simulink model "prob7_large_model"  (R2013a)
settings: Solver=ode45  StartTime=0.0  StopTime=0.5  RelTol=1e-3
libraries: fl_lib x10, nesl_utility x4
settings Model: Creator=Suddenlink  LastModifiedBy=Suddenlink

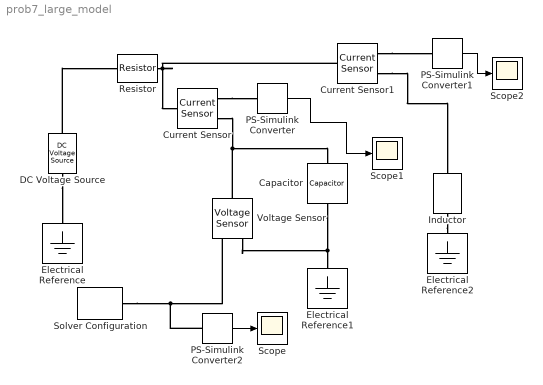
== system prob7_large_model ==
  Capacitor : fl_lib/Electrical/Electrical Elements/Capacitor  c=1e-6 F  v0=0 V  r=1e-6 Ohm  g=0 1/Ohm  i_Log=off  v_Log=off  vc_Log=off  LocalVarNames=|i|v|vc  LocalVarDescs=|i|v|Internal variable for voltage across capacitor term  LocalVarLogging=[0 0 0]
  Current Sensor : fl_lib/Electrical/Electrical Sensors/Current Sensor  i1_Log=off  v1_Log=off  LocalVarNames=|i1|v1  LocalVarDescs=|i1|v1  LocalVarLogging=[0 0]
  Current Sensor1 : fl_lib/Electrical/Electrical Sensors/Current Sensor  i1_Log=off  v1_Log=off  LocalVarNames=|i1|v1  LocalVarDescs=|i1|v1  LocalVarLogging=[0 0]
  DC Voltage Source : fl_lib/Electrical/Electrical Sources/DC Voltage Source  v0=1 V  i_Log=off  v_Log=off  LocalVarNames=|i|v  LocalVarDescs=|i|v  LocalVarLogging=[0 0]
  Electrical Reference : fl_lib/Electrical/Electrical Elements/Electrical Reference  i_Log=off  LocalVarNames=|i  LocalVarDescs=|i  LocalVarLogging=0
  Electrical Reference1 : fl_lib/Electrical/Electrical Elements/Electrical Reference  i_Log=off  LocalVarNames=|i  LocalVarDescs=|i  LocalVarLogging=0
  Electrical Reference2 : fl_lib/Electrical/Electrical Elements/Electrical Reference  i_Log=off  LocalVarNames=|i  LocalVarDescs=|i  LocalVarLogging=0
  Inductor : fl_lib/Electrical/Electrical Elements/Inductor  l=1e-6 H  i0=0 A  r=0 Ohm  g=1e-9 1/Ohm  i_Log=off  v_Log=off  i_L_Log=off  LocalVarNames=|i|v|i_L  LocalVarDescs=|i|v|Internal variable for current through inductor term  LocalVarLogging=[0 0 0]
  PS-Simulink Converter : nesl_utility/PS-Simulink Converter  PhysicalDomain=network_engine_domain  SubClassName=ps_output  LeftPortType=input  RightPortType=output  PseudoPeriodic=off  Frequencies=[]  Unit=1  AffineConversion=off
  PS-Simulink Converter1 : nesl_utility/PS-Simulink Converter  PhysicalDomain=network_engine_domain  SubClassName=ps_output  LeftPortType=input  RightPortType=output  PseudoPeriodic=off  Frequencies=[]  Unit=1  AffineConversion=off
  PS-Simulink Converter2 : nesl_utility/PS-Simulink Converter  PhysicalDomain=network_engine_domain  SubClassName=ps_output  LeftPortType=input  RightPortType=output  PseudoPeriodic=off  Frequencies=[]  Unit=1  AffineConversion=off
  Resistor : fl_lib/Electrical/Electrical Elements/Resistor  R=1 Ohm  i_Log=off  v_Log=off  LocalVarNames=|i|v  LocalVarDescs=|i|v  LocalVarLogging=[0 0]
  Scope : Scope
  Scope1 : Scope
  Scope2 : Scope
      settings: SaveName=ScopeData2
  Solver Configuration : nesl_utility/Solver Configuration  PhysicalDomain=network_engine_domain  SubClassName=solver  LeftPortType=input  RightPortType=generic  Accelerate=off  Tones=[]  Harmonics=[]  SimulateNoise=off  Profile=off  UseLocalSampling=off  EnableSwitchedLinearOptims=on  FrequencyDomain=off  UseCCode=off  UseNewInitialization=off  DoDC=off  ResidualTolerance=1e-09  UseLocalSolver=off  LocalSolverChoice=NE_BACKWARD_EULER_ADVANCER  LocalSolverSampleTime=0.001  DoFixedCost=off  MaxNonlinIter=3  MaxModeIter=2  LinearAlgebra=Sparse  DelaysMemoryBudget=1024
  Voltage Sensor : fl_lib/Electrical/Electrical Sensors/Voltage Sensor  i1_Log=off  v1_Log=off  LocalVarNames=|i1|v1  LocalVarDescs=|i1|v1  LocalVarLogging=[0 0]
  wires:
  PS-Simulink Converter2/1 -> Scope/1
  PS-Simulink Converter/1 -> Scope1/1
  PS-Simulink Converter1/1 -> Scope2/1
  connections:
  DC Voltage Source/RConn1 -- Electrical Reference/LConn1
  DC Voltage Source/LConn1 -- Resistor/LConn1
  Resistor/RConn1 -- Current Sensor/LConn1 -- Current Sensor1/LConn1
  Voltage Sensor/LConn1 -- Current Sensor/RConn2 -- Capacitor/LConn1
  Capacitor/RConn1 -- Voltage Sensor/RConn2 -- Electrical Reference1/LConn1
  Inductor/LConn1 -- Electrical Reference2/LConn1
  Solver Configuration/RConn1 -- PS-Simulink Converter2/LConn1 -- Voltage Sensor/RConn1
  Current Sensor/RConn1 -- PS-Simulink Converter/LConn1
  Current Sensor1/RConn1 -- PS-Simulink Converter1/LConn1
  Current Sensor1/RConn2 -- Inductor/RConn1
